simulink model "flyback"  (R2024b)
settings: Solver=ode23tb  StartTime=0.0  StopTime=0.104  MaxStep=1e-6  RelTol=1e-3
libraries: spsMeanLib x5, spsCurrentMeasurementLib x4, spsVoltageMeasurementLib x3, spsSeriesRLCBranchLib x2, spsDCVoltageSourceLib x1, spsDiodeLib x1, spsGroundLib x1, spsIGBTLib x1, spsLinearTransformerLib x1, spsRMSLib x1, sps_lib x1
settings Model: Creator=m_pek  LastModifiedBy=m_pek

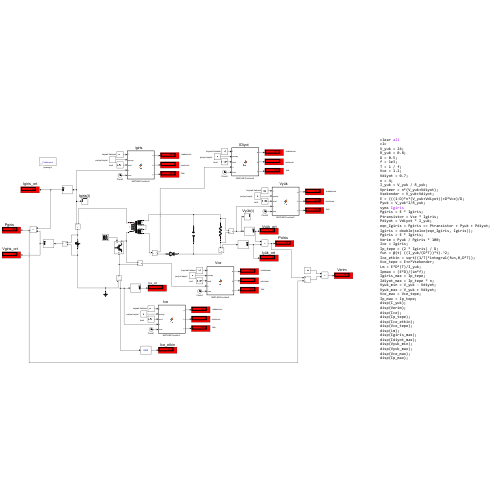
[thumbnail: Simulink's stored preview of the top-level diagram]
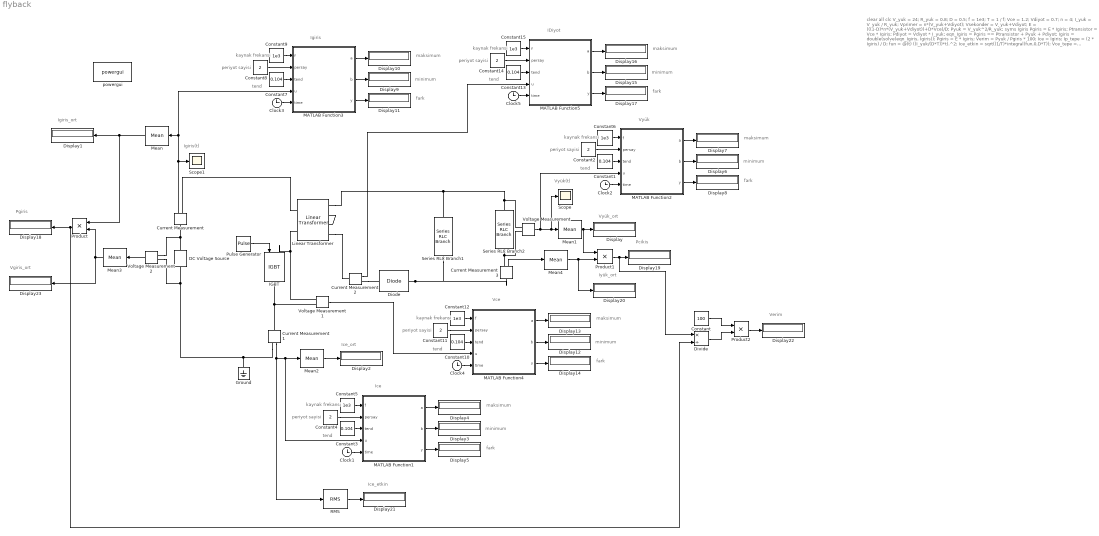
== system flyback ==
  note: clear all
      | clc
      | V_yuk = 24;
      | R_yuk = 0.8;
      | D = 0.5;
      | f = 1e3;
      | T = 1 / f;
      | Vce = 1.2;
      | Vdiyot = 0.7;
      | n = 4;
      | I_yuk = V_yuk / R_yuk;
      | Vprimer = n*(V_yuk+Vdiyot);
      | Vsekonder = V_yuk+Vdiyot;
      | E = (((1-D)*n*(V_yuk+Vdiyot))+D*Vce)/D;
      | Pyuk = V_yuk^2/R_yuk;
      | syms Igiris
      | Pgiris = E * Igiris;
      | Ptransistor = Vce * Igiris;
      | Pdiyot = Vdiyot * I_yuk;
      | eqn_Igiris = Pgiris == Ptransistor + Pyuk + Pdiyot;
      | Igiris = double(solve(eqn_Igiris, Igiris));
      | Pgiris = E * Igiris;
      | Verim = Pyuk / Pgiris * 100;
      | Ice = Igiris;
      | Ip_tepe = (2 * Igiris) / D;
      | fun = @(t) ((I_yuk/(D*T))*t).^2;
      | Ice_etkin = sqrt((1/T)*integral(fun,0,D*T));
      | Vce_tepe = E+n*Vsekonder;
      | Lm = E*D*(T)/I_yuk;
      | Ipmax = (E*D)/(Lm*f);
      | Igiris_max = Ip_tepe;
      | Idiyot_max = Ip_tepe * n;
      | Vyuk_min = V_yuk - Vdiyot;
      | Vyuk_max = V_yuk + Vdiyot;
      | Vce_max = Vce_tepe;
      | Ip_max = Ip_tepe;
      | disp(I_yuk);
      | disp(Verim);
      | disp(Ice);
      | disp(Ip_tepe);
      | disp(Ice_etkin);
      | disp(Vce_tepe);
      | disp(Lm);
      | disp(Igiris_max);
      | disp(Idiyot_max);
      | disp(Vyuk_min);
      | disp(Vyuk_max);
      | disp(Vce_max);
      | disp(Ip_max);
  note: Ice_ort
  note: fark
  note: periyot sayisi
  note: maksimum
  note: minimum
  note: kaynak frekansi
  note: tend
  note: Ice
  note: fark
  note: periyot sayisi
  note: maksimum
  note: minimum
  note: kaynak frekansi
  note: tend
  note: Vyük
  note: fark
  note: periyot sayisi
  note: maksimum
  note: minimum
  note: kaynak frekansi
  note: tend
  note: Igiris
  note: fark
  note: periyot sayisi
  note: maksimum
  note: minimum
  note: kaynak frekansi
  note: tend
  note: Vce
  note: fark
  note: periyot sayisi
  note: maksimum
  note: minimum
  note: kaynak frekansi
  note: tend
  note: IDiyot
  note: Vyük_ort
  note: Ice_etkin
  note: Verim
  note: Pcikis
  note: Iyük_ort
  note: Vgiris_ort
  note: Pgiris
  note: Vyük(t)
  note: Igiris(t)
  note: Igiris_ort
  Clock{1..5} (5 alike) : Clock
      settings: Decimation=100
  Constant : Constant  Value=100
  Constant{1,3,7,10,13} (5 alike) : Constant  Value=0.104  SampleTime=0
  Constant{2,4,8,11,14} (5 alike) : Constant  Value=2  SampleTime=0
  Constant{5..6,9,12,15} (5 alike) : Constant  Value=1e3  SampleTime=0
  Current Measurement{,1..3} (4 alike) : spsCurrentMeasurementLib/Current Measurement  PhasorSimulation=off  OutputType=Complex  PSBequivalent=0
  DC Voltage Source : spsDCVoltageSourceLib/DC Voltage Source  Amplitude=100  Measurements=None
  Diode : spsDiodeLib/Diode  Ron=1e-10  Lon=0  Vf=0.7  IC=0  UseSnubber=0  Rs=500  Cs=250e-9  Measurements=off
  Display{,1..23} (24 alike) : Display
  Divide : Product  Inputs=*/
  Ground : spsGroundLib/Ground  LConnTagsString=a
  IGBT : spsIGBTLib/IGBT  Ron=1e-8  Lon=0  Vf=1.2  Tf=1e-6  Tt=2e-6  IC=0  Rs=1e5  Cs=inf  Measurements=off
  Linear Transformer : spsLinearTransformerLib/Linear Transformer  UNITS=SI  NominalPower=[ 1000 50 ]  winding1=[100 0 0]  winding2=[12 0 0]  ThreeWindings=on  winding3=[12 0 0]  RmLm=[1e6 1.67e-3]  Measurements=None  DataType=on
  MATLAB Function1 : MATLAB Function  TreatAsAtomicUnit=on
  MATLAB Function2 : MATLAB Function  TreatAsAtomicUnit=on
  MATLAB Function3 : MATLAB Function  TreatAsAtomicUnit=on
  MATLAB Function4 : MATLAB Function  TreatAsAtomicUnit=on
  MATLAB Function5 : MATLAB Function  TreatAsAtomicUnit=on
  Mean{,1..4} (5 alike) : spsMeanLib/Mean  Freq=60  Vinit=0  Ts=0
  Product : Product
  Product1 : Product
  Product2 : Product
  Pulse Generator : DiscretePulseGenerator  PulseType=Time based  Period=1/1e3  PulseWidth=50
  RMS : spsRMSLib/RMS  TrueRMS=on  Freq=60  RMSInit=120  Ts=0
  Scope : Scope
  Scope1 : Scope
  Series RLC Branch1 : spsSeriesRLCBranchLib/Series RLC Branch  LConnTagsString=__new0  RConnTagsString=__new0  BranchType=C  Resistance=1  Inductance=1e-3  SetiL0=off  InitialCurrent=0  Capacitance=0.0405  Setx0=off  InitialVoltage=0  Measurements=None
  Series RLC Branch2 : spsSeriesRLCBranchLib/Series RLC Branch  LConnTagsString=__new0  RConnTagsString=__new0  BranchType=R  Resistance=0.8  Inductance=1e-3  SetiL0=off  InitialCurrent=0  Capacitance=1e-6  Setx0=off  InitialVoltage=0  Measurements=None
  Voltage Measurement : spsVoltageMeasurementLib/Voltage Measurement  PhasorSimulation=off  OutputType=Complex  PSBequivalent=0
  Voltage Measurement1 : spsVoltageMeasurementLib/Voltage Measurement  PhasorSimulation=off  OutputType=Complex  PSBequivalent=0
  Voltage Measurement2 : spsVoltageMeasurementLib/Voltage Measurement  PhasorSimulation=off  OutputType=Complex  PSBequivalent=0
  powergui : sps_lib/powergui  Priority=1  SimulationMode=Continuous  SampleTime=50e-6  frequency=60  Iterations=50  frequencyindice=0  Pbase=100e6  ErrMax=1e-4  UnitsV=kV  UnitsW=MW  buscounter=0  FunctionMessages=off  echomessages=off  EnableUseOfTLC=off  CurrentSourceSwitches=off  DisableSnubberDevices=on  DisableRonSwitches=off  DisableVfSwitches=off  DisplayEquations=off  AutomaticDiscreteSolvers=off  SolverType=Tustin/Backward Euler (TBE)  Interpol=off  ExternalGateDelay=off  methode=off  Ts=100  x0status=blocks  SPID=on  SwTol=0  HookPort=off  NonlinearTolerance=1e-4  nMaxIteration=100  ContinueOnMaxIteration=off  RestoreLinks=warning  ResistiveCurrentMeasurement=off  Frange=[0:2:500]  Ylog=off  Xlog=on  ShowGrid=off  save=off  variable=ZData  structure=0  ZoomFFT=off  StartTime=0.0  cycles=1  DisplayStyle=1  fundamental=60  FreqAxis=off  MaxFrequency=1000  frequencyindicesteady=1  RmsSteady=1  display=off
  wires:
  Pulse Generator/1 -> IGBT/1
  Mean/1 -> Display1/1, Product/1
  Mean1/1 -> Product1/1, Display/1
  Mean2/1 -> Display2/1
  Constant5/1 -> MATLAB Function1/1(f)
  MATLAB Function1/3(y) -> Display5/1
  MATLAB Function1/2(b) -> Display3/1
  Clock1/1 -> MATLAB Function1/5(time)
  MATLAB Function1/1(a) -> Display4/1
  Constant3/1 -> MATLAB Function1/3(tend)
  Constant4/1 -> MATLAB Function1/2(persay)
  Constant2/1 -> MATLAB Function2/2(persay)
  Constant1/1 -> MATLAB Function2/3(tend)
  MATLAB Function2/1(a) -> Display7/1
  Voltage Measurement/1 -> Scope/1, Mean1/1, MATLAB Function2/4(u)
  Clock2/1 -> MATLAB Function2/5(time)
  MATLAB Function2/2(b) -> Display6/1
  MATLAB Function2/3(y) -> Display8/1
  Constant6/1 -> MATLAB Function2/1(f)
  Constant9/1 -> MATLAB Function3/1(f)
  MATLAB Function3/3(y) -> Display11/1
  MATLAB Function3/2(b) -> Display9/1
  Clock3/1 -> MATLAB Function3/5(time)
  Current Measurement/1 -> Mean/1, MATLAB Function3/4(u), Scope1/1
  MATLAB Function3/1(a) -> Display10/1
  Constant7/1 -> MATLAB Function3/3(tend)
  Constant8/1 -> MATLAB Function3/2(persay)
  Constant11/1 -> MATLAB Function4/2(persay)
  Constant10/1 -> MATLAB Function4/3(tend)
  MATLAB Function4/1(a) -> Display13/1
  Voltage Measurement1/1 -> MATLAB Function4/4(u)
  Clock4/1 -> MATLAB Function4/5(time)
  MATLAB Function4/2(b) -> Display12/1
  MATLAB Function4/3(y) -> Display14/1
  Constant12/1 -> MATLAB Function4/1(f)
  Constant15/1 -> MATLAB Function5/1(f)
  MATLAB Function5/3(y) -> Display17/1
  MATLAB Function5/2(b) -> Display15/1
  Clock5/1 -> MATLAB Function5/5(time)
  Current Measurement2/1 -> MATLAB Function5/4(u)
  MATLAB Function5/1(a) -> Display16/1
  Constant13/1 -> MATLAB Function5/3(tend)
  Constant14/1 -> MATLAB Function5/2(persay)
  Current Measurement1/1 -> RMS/1, MATLAB Function1/4(u), Mean2/1
  Voltage Measurement2/1 -> Mean3/1
  Mean3/1 -> Display23/1, Product/2
  Product/1 -> Divide/2, Display18/1
  Current Measurement3/1 -> Mean4/1
  Mean4/1 -> Display20/1, Product1/2
  Product1/1 -> Divide/1, Display19/1
  RMS/1 -> Display21/1
  Product2/1 -> Display22/1
  Constant/1 -> Product2/1
  Divide/1 -> Product2/2
  connections:
  DC Voltage Source/RConn1 -- Current Measurement/LConn1 -- Voltage Measurement2/LConn1
  Linear Transformer/RConn4 -- Current Measurement2/LConn1
  Linear Transformer/RConn1 -- Series RLC Branch1/RConn1 -- Voltage Measurement/LConn2 -- Series RLC Branch2/RConn1
  Diode/RConn1 -- Current Measurement3/LConn1 -- Series RLC Branch1/LConn1
  IGBT/LConn1 -- Voltage Measurement1/LConn1 -- Linear Transformer/LConn2
  Voltage Measurement1/LConn2 -- Current Measurement1/LConn1 -- IGBT/RConn1
  Linear Transformer/RConn2 -- Linear Transformer/RConn3
  Current Measurement/RConn1 -- Linear Transformer/LConn1
  Ground/LConn1 -- Current Measurement1/RConn1 -- Voltage Measurement2/LConn2 -- DC Voltage Source/LConn1
  Current Measurement2/RConn1 -- Diode/LConn1
  Voltage Measurement/LConn1 -- Current Measurement3/RConn1 -- Series RLC Branch2/LConn1

== matlab function flyback/MATLAB Function1 ==
  settings: updateMethod=DISCRETE  sampleTime=50e-8
  data: a output; b output; f input; persay input; tend input; u input; y output; time input
function [a,b,y] = fcn(f,persay,tend,u,time)
% persistent değişken; değişken değerini kalıcı olarak tutar ve direk atama
% yapılmadıkça değişmez. Normal değişkenler fonksiyonun her yenilenme 
% durumunda sıfırlanırken, persistent değişkeni, kalıcı olması sebebiyle,
% bir önceki değeri tutabilme yeteneğine sahiptir. 
% Bu da bize bir önceki değer ile güncel değerinizi karşılaştırma olanağı
% sunar.
a=1/0;b=0;
persistent enbuyuk;
persistent enkucuk;
persistent fark;
% Eğer persistent değişkenini en başta persistent enbuyuk = 0; olarak 
% tanımlarsak, sürekli 0 olarak kalacaktır. Aynı zamanda eğer bir ilk değer 
% vermezseniz "null" değerini taşıyacağından, if yapılarında hata
% verecektir. Bu hatadan kaçınmak için, isempty komutu ile persistent
% değişkenlerinin "null" olup olmadığını kontrol edilir ve ilk değer ataması
% yapılır. Bu değişkenler sadece  fonksiyon ilk kez çalıştığında
% null olacağı için(daha sonra sürekli gelen değeri tuttuğu yukarıda söylenmişti)
% başlangıçta, bir kereye mahsus olarak,  aşağıdaki if yapısı doğrulanacak 
% ve değişkenlere ilk değerler atanacaktır.
%
if (isempty(enkucuk) || isempty(enbuyuk))  
enkucuk = 1/0;   
enbuyuk = 0;
end
if (time>tend-(persay+1)*1/f) && (time<=tend) % Periyot ~= 0.01 // Son iki periyodu hesaplar.
    if u >= enbuyuk
        enbuyuk = u;
     end
    if u < enkucuk   
        enkucuk = u;
    end
end
fark = enbuyuk - enkucuk;
a=enbuyuk;
b=enkucuk;
y=fark;
end

== matlab function flyback/MATLAB Function2 ==
  settings: updateMethod=DISCRETE  sampleTime=50e-8
  data: a output; b output; f input; persay input; tend input; u input; y output; time input
function [a,b,y] = fcn(f,persay,tend,u,time)
% persistent değişken; değişken değerini kalıcı olarak tutar ve direk atama
% yapılmadıkça değişmez. Normal değişkenler fonksiyonun her yenilenme 
% durumunda sıfırlanırken, persistent değişkeni, kalıcı olması sebebiyle,
% bir önceki değeri tutabilme yeteneğine sahiptir. 
% Bu da bize bir önceki değer ile güncel değerinizi karşılaştırma olanağı
% sunar.
a=1/0;b=0;
persistent enbuyuk;
persistent enkucuk;
persistent fark;
% Eğer persistent değişkenini en başta persistent enbuyuk = 0; olarak 
% tanımlarsak, sürekli 0 olarak kalacaktır. Aynı zamanda eğer bir ilk değer 
% vermezseniz "null" değerini taşıyacağından, if yapılarında hata
% verecektir. Bu hatadan kaçınmak için, isempty komutu ile persistent
% değişkenlerinin "null" olup olmadığını kontrol edilir ve ilk değer ataması
% yapılır. Bu değişkenler sadece  fonksiyon ilk kez çalıştığında
% null olacağı için(daha sonra sürekli gelen değeri tuttuğu yukarıda söylenmişti)
% başlangıçta, bir kereye mahsus olarak,  aşağıdaki if yapısı doğrulanacak 
% ve değişkenlere ilk değerler atanacaktır.
%
if (isempty(enkucuk) || isempty(enbuyuk))  
enkucuk = 1/0;   
enbuyuk = 0;
end
if (time>tend-(persay+1)*1/f) && (time<=tend) % Periyot ~= 0.01 // Son iki periyodu hesaplar.
    if u >= enbuyuk
        enbuyuk = u;
     end
    if u < enkucuk   
        enkucuk = u;
    end
end
fark = enbuyuk - enkucuk;
a=enbuyuk;
b=enkucuk;
y=fark;
end

== matlab function flyback/MATLAB Function3 ==
  settings: updateMethod=DISCRETE  sampleTime=50e-8
  data: a output; b output; f input; persay input; tend input; u input; y output; time input
function [a,b,y] = fcn(f,persay,tend,u,time)
% persistent değişken; değişken değerini kalıcı olarak tutar ve direk atama
% yapılmadıkça değişmez. Normal değişkenler fonksiyonun her yenilenme 
% durumunda sıfırlanırken, persistent değişkeni, kalıcı olması sebebiyle,
% bir önceki değeri tutabilme yeteneğine sahiptir. 
% Bu da bize bir önceki değer ile güncel değerinizi karşılaştırma olanağı
% sunar.
a=1/0;b=0;
persistent enbuyuk;
persistent enkucuk;
persistent fark;
% Eğer persistent değişkenini en başta persistent enbuyuk = 0; olarak 
% tanımlarsak, sürekli 0 olarak kalacaktır. Aynı zamanda eğer bir ilk değer 
% vermezseniz "null" değerini taşıyacağından, if yapılarında hata
% verecektir. Bu hatadan kaçınmak için, isempty komutu ile persistent
% değişkenlerinin "null" olup olmadığını kontrol edilir ve ilk değer ataması
% yapılır. Bu değişkenler sadece  fonksiyon ilk kez çalıştığında
% null olacağı için(daha sonra sürekli gelen değeri tuttuğu yukarıda söylenmişti)
% başlangıçta, bir kereye mahsus olarak,  aşağıdaki if yapısı doğrulanacak 
% ve değişkenlere ilk değerler atanacaktır.
%
if (isempty(enkucuk) || isempty(enbuyuk))  
enkucuk = 1/0;   
enbuyuk = 0;
end
if (time>tend-(persay+1)*1/f) && (time<=tend) % Periyot ~= 0.01 // Son iki periyodu hesaplar.
    if u >= enbuyuk
        enbuyuk = u;
     end
    if u < enkucuk   
        enkucuk = u;
    end
end
fark = enbuyuk - enkucuk;
a=enbuyuk;
b=enkucuk;
y=fark;
end

== matlab function flyback/MATLAB Function4 ==
  settings: updateMethod=DISCRETE  sampleTime=50e-8
  data: a output; b output; f input; persay input; tend input; u input; y output; time input
function [a,b,y] = fcn(f,persay,tend,u,time)
% persistent değişken; değişken değerini kalıcı olarak tutar ve direk atama
% yapılmadıkça değişmez. Normal değişkenler fonksiyonun her yenilenme 
% durumunda sıfırlanırken, persistent değişkeni, kalıcı olması sebebiyle,
% bir önceki değeri tutabilme yeteneğine sahiptir. 
% Bu da bize bir önceki değer ile güncel değerinizi karşılaştırma olanağı
% sunar.
a=1/0;b=0;
persistent enbuyuk;
persistent enkucuk;
persistent fark;
% Eğer persistent değişkenini en başta persistent enbuyuk = 0; olarak 
% tanımlarsak, sürekli 0 olarak kalacaktır. Aynı zamanda eğer bir ilk değer 
% vermezseniz "null" değerini taşıyacağından, if yapılarında hata
% verecektir. Bu hatadan kaçınmak için, isempty komutu ile persistent
% değişkenlerinin "null" olup olmadığını kontrol edilir ve ilk değer ataması
% yapılır. Bu değişkenler sadece  fonksiyon ilk kez çalıştığında
% null olacağı için(daha sonra sürekli gelen değeri tuttuğu yukarıda söylenmişti)
% başlangıçta, bir kereye mahsus olarak,  aşağıdaki if yapısı doğrulanacak 
% ve değişkenlere ilk değerler atanacaktır.
%
if (isempty(enkucuk) || isempty(enbuyuk))  
enkucuk = 1/0;   
enbuyuk = 0;
end
if (time>tend-(persay+1)*1/f) && (time<=tend) % Periyot ~= 0.01 // Son iki periyodu hesaplar.
    if u >= enbuyuk
        enbuyuk = u;
     end
    if u < enkucuk   
        enkucuk = u;
    end
end
fark = enbuyuk - enkucuk;
a=enbuyuk;
b=enkucuk;
y=fark;
end

== matlab function flyback/MATLAB Function5 ==
  settings: updateMethod=DISCRETE  sampleTime=50e-8
  data: a output; b output; f input; persay input; tend input; u input; y output; time input
function [a,b,y] = fcn(f,persay,tend,u,time)
% persistent değişken; değişken değerini kalıcı olarak tutar ve direk atama
% yapılmadıkça değişmez. Normal değişkenler fonksiyonun her yenilenme 
% durumunda sıfırlanırken, persistent değişkeni, kalıcı olması sebebiyle,
% bir önceki değeri tutabilme yeteneğine sahiptir. 
% Bu da bize bir önceki değer ile güncel değerinizi karşılaştırma olanağı
% sunar.
a=1/0;b=0;
persistent enbuyuk;
persistent enkucuk;
persistent fark;
% Eğer persistent değişkenini en başta persistent enbuyuk = 0; olarak 
% tanımlarsak, sürekli 0 olarak kalacaktır. Aynı zamanda eğer bir ilk değer 
% vermezseniz "null" değerini taşıyacağından, if yapılarında hata
% verecektir. Bu hatadan kaçınmak için, isempty komutu ile persistent
% değişkenlerinin "null" olup olmadığını kontrol edilir ve ilk değer ataması
% yapılır. Bu değişkenler sadece  fonksiyon ilk kez çalıştığında
% null olacağı için(daha sonra sürekli gelen değeri tuttuğu yukarıda söylenmişti)
% başlangıçta, bir kereye mahsus olarak,  aşağıdaki if yapısı doğrulanacak 
% ve değişkenlere ilk değerler atanacaktır.
%
if (isempty(enkucuk) || isempty(enbuyuk))  
enkucuk = 1/0;   
enbuyuk = 0;
end
if (time>tend-(persay+1)*1/f) && (time<=tend) % Periyot ~= 0.01 // Son iki periyodu hesaplar.
    if u >= enbuyuk
        enbuyuk = u;
     end
    if u < enkucuk   
        enkucuk = u;
    end
end
fark = enbuyuk - enkucuk;
a=enbuyuk;
b=enkucuk;
y=fark;
end
